simulink library "InertialPointing"  (R2014b)
settings: Solver=VariableStepAuto  StartTime=0.0  StopTime=10.0  RelTol=1e-3
undefined symbols (not defined in the file or in its folder): ConfParam
settings Model: Creator=y.akisheva  LastModifiedBy=Hp
settings DataIOCC: SaveFormat=Dataset
settings OptimizationCC: UseDivisionForNetSlopeComputation=off  SimCompilerOptimization=off
settings DebuggingCC: SolverPrmCheckMsg=none  FrameProcessingCompatibilityMsg=error  AllowSymbolicDim=off
settings HardwareCC: ProdBitPerPointer=64  ProdLargestAtomicFloat=Float  ProdIntDivRoundTo=Zero  ProdEndianess=LittleEndian  ProdWordSize=64  ProdHWDeviceType=Intel->x86-64 (Windows64)
settings RTWCC: RTWCompilerOptimization=off
settings GRTTargetCC: GeneratePreprocessorConditionals=Use local settings
settings ConfigComp: CovMetricSettings=dw  CovHtmlReporting=on  CovSaveCumulativeToWorkspaceVar=on  CovSaveSingleToWorkspaceVar=on  CovExternalEMLEnable=off

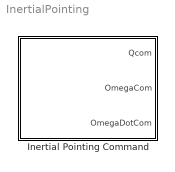
== system InertialPointing ==
  Inertial Pointing Command : Subsystem

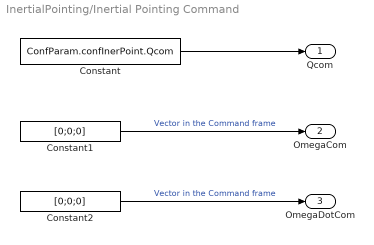
== system InertialPointing/Inertial Pointing Command ==
  Constant : Constant  Value=ConfParam.confInerPoint.Qcom
  Constant1 : Constant  Value=[0;0;0]
  Constant2 : Constant  Value=[0;0;0]
  Qcom : Outport
  OmegaCom : Outport  Port=2
  OmegaDotCom : Outport  Port=3
  wires:
  Constant1/1 -> OmegaCom/1  "Vector in the Command frame"
  Constant2/1 -> OmegaDotCom/1  "Vector in the Command frame"
  Constant/1 -> Qcom/1
